simulink model "EVX_Lap_Simulation 2"  (R2018b)
settings: Solver=FixedStepAuto  StartTime=0  StopTime=120  FixedStep=0.001  MaxStep=0.01  RelTol=1e-2
values from neighbouring files (symbols this model uses):
  velocity_dnew = velocity_d + 0.4 .* (velocity_dmax - velocity_d)    [Run_Sim(with_fmincon).m]
undefined symbols (not defined in the file or in its folder): dist, theta_d
libraries: simulink x1
(part 3 of 3)

== matlab function EVX_Lap_Simulation 2/EVX_Vehicle_Model/Car_Parameters/MATLAB Function20 ==
  data: Fzo output; Ro output; q_Bz1 output; q_Bz2 output; q_Bz3 output; q_Bz4 output; q_Bz5 output; q_Bz9 output; q_Bz10 output; q_Cz1 output; q_Dz1 output; q_Dz2 output; q_Dz3 output; q_Dz4 output; q_Dz6 output; q_Dz7 output; q_Dz8 output; q_Dz9 output; q_Ez1 output; q_Ez2 output; q_Ez3 output; q_Ez4 output; q_Ez5 output; q_Hz1 output; q_Hz2 output; q_Hz3 output; q_Hz4 output; p_Cy1 output; p_Dy1 output; p_Dy2 output; p_Dy3 output; p_Ey1 output; p_Ey2 output; p_Ey3 output; p_Ey4 output; p_Ky1 output; p_Ky2 output; p_Ky3 output; p_Hy1 output; p_Hy2 output; p_Hy3 output; p_Vy1 output; p_Vy2 output; p_Vy3 output; p_Vy4 output; p_Cx1 output; p_Dx1 output; p_Dx2 output; p_Ex1 output; p_Ex2 output; p_Ex3 output; p_Ex4 output; p_Kx1 output; p_Kx2 output; p_Kx3 output; p_Hx1 output; p_Hx2 output; p_Vx1 output; p_Vx2 output
function [Fzo,Ro,q_Bz1,q_Bz2,q_Bz3,q_Bz4,q_Bz5,q_Bz9,q_Bz10,q_Cz1,q_Dz1,...
    q_Dz2,q_Dz3,q_Dz4,q_Dz6,q_Dz7,q_Dz8,q_Dz9,q_Ez1,q_Ez2,q_Ez3,q_Ez4,q_Ez5,...
    q_Hz1,q_Hz2,q_Hz3,q_Hz4,p_Cy1,p_Dy1,p_Dy2,p_Dy3,p_Ey1,p_Ey2,p_Ey3,...
    p_Ey4,p_Ky1,p_Ky2,p_Ky3,p_Hy1,p_Hy2,p_Hy3,p_Vy1,p_Vy2,p_Vy3,p_Vy4,...
    p_Cx1,p_Dx1,p_Dx2,p_Ex1,p_Ex2,p_Ex3,p_Ex4,p_Kx1,p_Kx2,p_Kx3,p_Hx1,...
    p_Hx2,p_Vx1,p_Vx2] = Avon_FITO9241
% pacejka model coefficients provided by Stackpole Engineering Services
% for Avon tyre model FITO 9241
% as found in the document 'SES_FSAE_Tiredata_Rev3'
% Specs:
% Size	6.2/20-13
% Pressure 12 psi


Fzo =	1122.74; % N
Ro = 0.25400; % m

% [ALIGNING COEFFICIENTS]
q_Bz1 =	6.11547;
q_Bz2 =	-1.96461;
q_Bz3 =	1.02155;
q_Bz4 =	5.41323;
q_Bz5 =	-7.58049;
q_Bz9 =	0;
q_Bz10 = 0;
q_Cz1 =	1.25000;
q_Dz1 =	0.15275;
q_Dz2 =	-0.00637;
q_Dz3 =	-0.21282;
q_Dz4 =	0.02719;
q_Dz6 =	-0.00145;
q_Dz7 =	0.01039;
q_Dz8 =	-1.03566;
q_Dz9 =	0.24508;
q_Ez1 =	-4.00001;
q_Ez2 =	0;
q_Ez3 =	0.00003;
q_Ez4 =	0.29616;
q_Ez5 =	2.43287;
q_Hz1 =	-0.00124;
q_Hz2 =	-0.00769;
q_Hz3 =	0.49190;
q_Hz4 =	0.13660;

%  [LATERAL COEFFICIENTS]
p_Cy1 =	0.95232;
p_Dy1 =	2.65462;
p_Dy2 =	0.05198;
p_Dy3 =	-13.51679;
p_Ey1 =	0.29170;
p_Ey2 =	0.30617;
p_Ey3 =	-0.53331;
p_Ey4 =	1.52410;
p_Ky1 =	-27.31900;
p_Ky2 =	-1.06469;
p_Ky3 =	2.27460;
p_Hy1 =	0.00227;
p_Hy2 =	-0.00772;
p_Hy3 =	-0.12814;
p_Vy1 =	0.14237;
p_Vy2 =	-0.17287;
p_Vy3 =	-1.49583;
p_Vy4 =	4.55061;

% [LONGITUDINAL COEFFICIENTS]
p_Cx1 = 1.43990;
p_Dx1 =	2.59060;
p_Dx2 =	-0.36627;
p_Ex1 =	-0.24355;
p_Ex2 =	-0.66953;
p_Ex3 =	-3.71110;
p_Ex4 =	0.37836;
p_Kx1 =	36.76960;
p_Kx2 =	-23.37320;
p_Kx3 =	-0.45230;
p_Hx1 =	0.00098;
p_Hx2 =	0.00014;
p_Vx1 =	-0.04913;
p_Vx2 =	0.02482;

== matlab function EVX_Lap_Simulation 2/EVX_Vehicle_Model/Subsystem1/MATLAB Function8 ==
  data: Fz input; Fxo output; kappa input; alpha input; gam input; Fzo input; Ro input; Fyo output; Mzo output; q_Bz1 input; q_Bz2 input; q_Bz3 input; q_Bz4 input; q_Bz5 input; q_Bz9 input; q_Bz10 input; q_Cz1 input; q_Dz1 input; q_Dz2 input; q_Dz3 input; q_Dz4 input; q_Dz6 input; q_Dz7 input; q_Dz8 input; q_Dz9 input; q_Ez1 input; q_Ez2 input; q_Ez3 input; q_Ez4 input; q_Ez5 input; q_Hz1 input; q_Hz2 input; q_Hz3 input; q_Hz4 input; p_Cy1 input; p_Dy1 input; p_Dy2 input; p_Dy3 input; p_Ey1 input; p_Ey2 input; p_Ey3 input; p_Ey4 input; p_Ky1 input; p_Ky2 input; p_Ky3 input; p_Hy1 input; p_Hy2 input; p_Hy3 input; p_Vy1 input; p_Vy2 input; p_Vy3 input; p_Vy4 input; p_Cx1 input; p_Dx1 input; p_Dx2 input; p_Ex1 input; p_Ex2 input; p_Ex3 input; p_Ex4 input; p_Kx1 input; p_Kx2 input; p_Kx3 input; p_Hx1 input; p_Hx2 input; p_Vx1 input; p_Vx2 input; car_mu_scaling input; run_info input
function [Fxo,Fyo,Mzo] = Pacejka_Tyre_Model(Fz,kappa,alpha,gam,Fzo,Ro,...
    q_Bz1,q_Bz2,q_Bz3,q_Bz4,q_Bz5,q_Bz9,q_Bz10,q_Cz1,q_Dz1,...
    q_Dz2,q_Dz3,q_Dz4,q_Dz6,q_Dz7,q_Dz8,q_Dz9,q_Ez1,q_Ez2,q_Ez3,q_Ez4,q_Ez5,...
    q_Hz1,q_Hz2,q_Hz3,q_Hz4,p_Cy1,p_Dy1,p_Dy2,p_Dy3,p_Ey1,p_Ey2,p_Ey3,...
    p_Ey4,p_Ky1,p_Ky2,p_Ky3,p_Hy1,p_Hy2,p_Hy3,p_Vy1,p_Vy2,p_Vy3,p_Vy4,...
    p_Cx1,p_Dx1,p_Dx2,p_Ex1,p_Ex2,p_Ex3,p_Ex4,p_Kx1,p_Kx2,p_Kx3,p_Hx1,...
    p_Hx2,p_Vx1,p_Vx2,car_mu_scaling,run_info)
% Pacejka '96 tyre model
%
% Inputs:
% Fz:       normal force (N)
% kappa:    slip ratio (% between -1 and 1) +ve is driving, -ve is braking
% alpha:    slip angle (rad) +ve alpha generates +ve Fyo
% gam:      inclanation angle/camber (rad) +ve indicates top of tyre tipped
%           right
% Outputs:
% Fxo:      Longitudinal force (N)
% Fyo:      Lateral force (N)
% Mzo:      Aligning moment (Nm)


%% tyre coefficients
% each different type of tyre holds different scaling coefficients, load 
% these here Also loaded are unloaded tyre radius and nominal wheel load

% unpack the structure holding the coefficients
% Get the field names of the structure
% fields = fieldnames(carpacejka_coefs, '-full');

% for ii = 1:length(fields)
%     thisField = fields{ii};
%     create_variable = sprintf('%s = carpacejka_coefs%s;', thisField, thisField);
%     eval(create_variable);
% end
% clear('ii', 'thisField');
% clear('fields', 'create_variable');

%% register track conditions
% scaling factors affected by wet/dry conditions

    lambda_mux = 1; % peak friction coefficient
    lambda_muy = 1; % peak friction coefficient

% modify with user scaling factor
lambda_mux = lambda_mux*car_mu_scaling;
lambda_muy = lambda_muy*car_mu_scaling;

%% scaling factors
% default values for these values is 1 (except lambda_muV=0)
lambda_Fzo = 1; % nominal rated load
lambda_muV = 0; % with slip speed Vx decaying friction
lambda_Kx = 1; % brake slip stiffness
lambda_Ky = 1; % cornering stiffness
lambda_Cx = 1; % shape factor
lambda_Cy = 1; % shape factor
lambda_Ex = 1; % curvature factor
lambda_Ey = 1; % curvature factor
lambda_Hx = 1; % horizontal shift
lambda_Hy = 1; % horizontal shift
lambda_Vx = 1; % vertical shift
lambda_Vy = 1; % vertical shift
lambda_Kygam = 1; % camber force stiffness
lambda_Kzgam = 1; % camber torque stiffness
lambda_t = 1; % pneumatic trail
lambda_Mr = 1; % residual torque
lambda_ygam = 1;

if ~isrow(kappa) || ~isrow(alpha) || ~isrow(gam)
    kappa = transpose(kappa);
    alpha = transpose(alpha);
    gam = transpose(gam);
end

for ii=1:length(Fz)
    %% derived inputs
    dfz = (Fz(ii)-Fzo)/Fzo; % normalised change in vertical load
    
    %% longitudinal force (pure longitudinal slip)
    S_Vx = Fz(ii)*(p_Vx1+p_Vx2*dfz)*lambda_Vx*lambda_mux;
    S_Hx = (p_Hx1+p_Hx2*dfz)*lambda_Hx;
    kappa_x = kappa + S_Hx;
    K_xk = Fz(ii)*(p_Kx1+p_Kx2*dfz)*exp(-p_Kx3*dfz)*lambda_Kx;
    E_x = (p_Ex1+p_Ex2*dfz+p_Ex3*dfz^2)*(1-p_Ex4*sign(kappa_x))*lambda_Ex;
    mu_x = (p_Dx1+p_Dx2*dfz)*lambda_mux;
    D_x = mu_x*Fz(ii);
    C_x = p_Cx1*lambda_Cx;
    B_x = K_xk/(C_x*D_x);
    Fxo = D_x*sin(C_x*atan(B_x*kappa_x - E_x*(B_x*kappa_x-atan(B_x*kappa_x)))) + S_Vx;
    
    %% lateral force (pure lateral slip)
    gam_y = gam*lambda_ygam;
    C_y = p_Cy1*lambda_Cy;
    mu_y = (p_Dy1+p_Dy2*dfz)*(1-p_Dy3*gam^2)*lambda_muy;
    D_y = mu_y*Fz(ii);
    S_Hy = (p_Hy1+p_Hy2*dfz+p_Hy3*gam)*lambda_Hy;
    alpha_y = alpha + S_Hy;
    E_y = (p_Ey1+p_Ey2*dfz)*(1-(p_Ey3+p_Ey4*gam_y)*sign(alpha_y))*lambda_Ey;
    K_ya = p_Ky1*Fzo*sin(2*atan(Fz(ii)/(p_Ky2*Fzo*lambda_Fzo)))*(1-p_Ky3*abs(gam))*lambda_Fzo*lambda_Ky;
    B_y = K_ya/(C_y*D_y);
    S_Vy = Fz(ii)*((p_Vy1+p_Vy2*dfz)+(p_Vy3+p_Vy4*dfz)*gam*lambda_Vy*lambda_Kygam);
    Fyo = D_y*sin(C_y*atan(B_y*alpha_y - E_y*(B_y*alpha_y-atan(B_y*alpha_y)))) + S_Vy;
    
    %% aligning torque (pure side slip)
    B_t = (q_Bz1+q_Bz2*dfz+q_Bz3*dfz^2)*(1+q_Bz4*gam*q_Bz5*abs(gam))*lambda_Ky/lambda_muy;
    C_t = q_Cz1;
    D_t = (q_Dz1+q_Dz2*dfz)*(1+q_Dz3*gam+q_Dz4*gam^2)*Ro*lambda_t/Fzo;
    S_Ht = q_Hz1+q_Hz2*dfz+(q_Hz3+q_Hz4*dfz)*gam;
    alpha_t = alpha + S_Ht;
    E_t = (q_Ez1+q_Ez2*dfz+q_Ez3*dfz^2)*(1+(q_Ez4+q_Ez5*gam)*atan(B_t*C_t*alpha_t));
    B_r = (q_Bz9*lambda_Ky/lambda_muy+q_Bz10*B_y*C_y);
    D_r = Fz(ii)*((q_Dz6+q_Dz7*dfz)+(q_Dz8+q_Dz9*dfz)*gam)*Ro*lambda_muy*lambda_Mr;
    S_Hf = S_Hy + S_Vy/K_ya;
    alpha_r = alpha + S_Hf;
    Mzr = D_r*cos(atan(B_r*alpha_r))*cos(alpha);
    t = D_t*cos(C_t*atan(B_t*alpha_t-E_t*(B_t*alpha_t-atan(B_t*alpha_t))))*cos(alpha);
    Mzo = -t*Fyo + Mzr;
    
end

== matlab function EVX_Lap_Simulation 2/EVX_Vehicle_Model/Subsystem1/MATLAB Function ==
  data: x input; F_z output; xdot input; k input; c input
function F_z = fcn(x,xdot,k,c)

F_z = k * x + c * xdot;

== matlab function EVX_Lap_Simulation 2/EVX_Vehicle_Model/Car_Parameters/MATLAB Function21 ==
  data: whatever input; k_SFR output; Owen input; wants input; k_SFL output; k_SRR output; k_SRL output; c_SFR output; c_SFL output; c_SRR output; c_SRL output; k_TFR output; k_TFL output; k_TRR output; k_TRL output; c_TFR output; c_TFL output; c_TRR output; c_TRL output; k_RF output; k_RR output; k_FRIC output; c_RF output; c_RR output; c_FRIC output; gamma_FR output; gamma_FL output; gamma_RR output; gamma_RL output; I_WFR output; I_WFL output; I_WRR output; I_WRL output
function [k_SFR,k_SFL,k_SRR,k_SRL,c_SFR,c_SFL,c_SRR,c_SRL,k_TFR,k_TFL,...
    k_TRR,k_TRL,c_TFR,c_TFL,c_TRR,c_TRL,k_RF,k_RR,k_FRIC,c_RF,c_RR,...
    c_FRIC,gamma_FR,gamma_FL,gamma_RR,gamma_RL,I_WFR,I_WFL,I_WRR,I_WRL]...
    = Suspension_Mapping(whatever,Owen,wants)

% Suspension Stifnesses
k_SFR = 8000; %suspension stiffness front right (N/m)
k_SFL = 8000; %suspension stiffness front left (N/m)
k_SRR = 8000; %suspension stiffness rear right (N/m)
k_SRL = 8000; %suspension stiffness rear left (N/m)

% Tire Stifnesses
k_TFR = 10000; %tire stiffness front right (N/m)
k_TFL = 10000; %tire stiffness front left (N/m)
k_TRR = 10000; %tire stiffness rear right (N/m)
k_TRL = 10000; %tire stiffness rear left (N/m)

% Suspension Damping Coefficients
c_SFR = 1000; %suspension damping coefficient front right (Ns/m)
c_SFL = 1000; %suspension damping coefficient front left (Ns/m)
c_SRR = 1000; %suspension damping coefficientv rear right (Ns/m)
c_SRL = 1000; %suspension damping coefficient rear left (Ns/m)

% Tire Damping Coefficients
c_TFR = 2000; %tire damping coefficient front right (Ns/m)
c_TFL = 2000; %tire damping coefficient front left (Ns/m)
c_TRR = 2000; %tire damping coefficientv rear right (Ns/m)
c_TRL = 2000; %tire damping coefficient rear left (Ns/m)

% Roll Bar Stiffnesses
k_RF = 0; %front
k_RR = 0; %rear
k_FRIC = 0; %front to rear

% Roll Bar Damping
c_RF = 0; %front
c_RR = 0; %rear
c_FRIC = 0; %front to rear

% Camber (deg) (tilt right positive)
gamma_FRd = 0;
gamma_FLd = 0;
gamma_RRd = 0;
gamma_RLd = 0;

% Camber (Rad)
Deg2Rad = 0.0174533;
gamma_FR = gamma_FRd * Deg2Rad;
gamma_FL = gamma_FLd * Deg2Rad;
gamma_RR = gamma_RRd * Deg2Rad;
gamma_RL = gamma_RLd * Deg2Rad;

% Wheel Inertias
I_WFR = 2;
I_WFL = 2;
I_WRR = 2;
I_WRL = 2;

== matlab function EVX_Lap_Simulation 2/EVX_Vehicle_Model/MATLAB Function22 ==
  data: g output
function g  = Environment_Parameters

g = 9.81;

== matlab function EVX_Lap_Simulation 2/EVX_Vehicle_Model/Chassis Vertical Dynamics/MATLAB Function22 ==
  data: g input; F_zWFR output; m_WFR input; m_WFL input; m_WRR input; m_WRL input; F_zWFL output; F_zWRR output; F_zWRL output
function [F_zWFR,F_zWFL,F_zWRR,F_zWRL] = fcn(g,m_WFR,m_WFL,m_WRR,m_WRL)

F_zWFR = -g * m_WFR;
F_zWFL = -g * m_WFL;
F_zWRR = -g * m_WRR;
F_zWRL = -g * m_WRL;

== matlab function EVX_Lap_Simulation 2/EVX_Vehicle_Model/MATLAB Function23 ==
  data: v_y input; ratio_FR output; angle_FR output; ratio_FL output; angle_FL output; ratio_RR output; angle_RR output; ratio_RL output; angle_RL output; v_x input; a input; b input; d_F input; e_F input; d_R input; e_R input; Idot_z input; r_FR input; r_FL input; r_RR input; r_RL input; S_FR input; S_FL input; S_RR input; S_RL input; w_FR input; w_FL input; w_RR input; w_RL input
function [ratio_FR,angle_FR,ratio_FL,angle_FL,ratio_RR,angle_RR,ratio_RL,...
    angle_RL] = Tyre_Slips(v_y,v_x,a,b,d_F,e_F,d_R,e_R,Idot_z,r_FR,r_FL,...
    r_RR,r_RL,S_FR,S_FL,S_RR,S_RL,w_FR,w_FL,w_RR,w_RL)

beta = atan(v_y/v_x);

v_yFR = v_y + Idot_z * a;
v_yFL = v_y + Idot_z * a;
v_yRR = v_y + Idot_z * -b;
v_yRL = v_y + Idot_z * -b;

v_xFR = v_x - Idot_z * e_F;
v_xFL = v_x - Idot_z * -d_F;
v_xRR = v_x - Idot_z * e_R;
v_xRL = v_x - Idot_z * -d_R;

beta_FR = atan(v_yFR/v_xFR);
beta_FL = atan(v_yFL/v_xFL);
beta_RR = atan(v_yRR/v_xRR);
beta_RL = atan(v_yRL/v_xRL);

w0_FR = v_x / r_FR;
w0_FL = v_x / r_FL;
w0_RR = v_x / r_RR;
w0_RL = v_x / r_RL;

ratio_FR = (w_FR - w0_FR)/w0_FR;
angle_FR = beta_FR - S_FR;
ratio_FL = (w_FL - w0_FL)/w0_FL;
angle_FL = beta_FL - S_FL;
ratio_RR = (w_RR - w0_RR)/w0_RR;
angle_RR = beta_RR - S_RR;
ratio_RL = (w_RL - w0_RL)/w0_RL;
angle_RL = beta_RL - S_RL;

% ratio_FR = 0;
% angle_FR = 0;
% ratio_FL = 0;
% angle_FL = 0;
% ratio_RR = 0;
% angle_RR = 0;
% ratio_RL = 0;
% angle_RL = 0;

== matlab function EVX_Lap_Simulation 2/EVX_Vehicle_Model/Aero Model/MATLAB Function ==
  data: v_x input; F_d output
function F_d = Drag(v_x)

F_d = v_x * 10;

== matlab function EVX_Lap_Simulation 2/EVX_Vehicle_Model/Tyre Model/Pacejka Tyre Model/MATLAB Function5 ==
  data: SA input; F_y output; SL input; Fz input; F_x output; M_z output
function [F_y,F_x,M_z] = Pacejka4(SA,SL,Fz)
x1  =  0.0174533 .* SA;  %Slip
x2  = Fz;  % Fz
x3  =  150 * 0.0174533 .* SL;  %Slip ratio, with fudge factor
P = [2 1 12.5 1.55]; %Fitted to FSAE TTC Round 6 Run 2
D1  = P(1);
D2  = P(2);
B   = P(3);
C   = P(4);
D   = (D1 + D2/1000 .* x2) .* x2;   % peak value (normalized)
F_y  = D .* sin(C .* atan(B .* x1));
F_x  = D .*sin (C .* atan(B .* x3));
M_z = [0 0 0 0];

== matlab function EVX_Lap_Simulation 2/EVX_Vehicle_Model/Aero Model/MATLAB Function1 ==
  data: v_x input; F_z output
function F_z = Drag(v_x)

F_z = v_x * 2;

== matlab function EVX_Lap_Simulation 2/EVX_Vehicle_Model/Tyre Model/MATLAB Function1 ==
  data: x_W input; F_zT output; xdot_W input; k_T input; c_T input
function F_zT  = fcn(x_W,xdot_W,k_T,c_T)

F_zT = k_T .* (-x_W) + c_T .* (-xdot_W);

== matlab function EVX_Lap_Simulation 2/EVX Vehicle Model V2/Vertical Dynamics/8DOF Vibrations ==
  data: V input; A output; V output; D input; F input; zB input; dzB input; D output; w input; m input; I input; kc input; cc input; kt input; ks input; kr input; ct input; cs input; cr input; kt output; ct output
function [A,V,D,kt,ct] =   DOF_Dynamics(V,D,F,zB,dzB,w,m,I,kc,cc,kt,ks,kr,ct,cs,cr)

% Tyre Stifness = 0 when off ground
for i = 1:4
    if D(i) - zB(i) > 0
        kt(i) = 0;
        ct(i) = 0;
    end
end

% Wheel Positions
x_wFL = w(1,1);
x_wFR = w(1,2);
x_wRL = w(1,3);
x_wRR = w(1,4);

y_wFL = w(2,1);
y_wFR = w(2,2);
y_wRL = w(2,3);
y_wRR = w(2,4);

% Chassis Forces
Fw_FL = F(1);
Fw_FR = F(2);
Fw_RL = F(3);
Fw_RR = F(4);
Fc_z = F(5);
Mc_y = F(6);
McF_x = F(7);
McR_x = F(8);

% Mass & Intertias
m_WFL = m(1);
m_WFR = m(2);
m_WRL = m(3);
m_WRR = m(4);
m_c = m(5);
I_cy = I(1);
I_xF = I(2);
I_xR = I(3);
I_z = I(4);

% Base Displacements
zB_FL = zB(1);
zB_FR = zB(2);
zB_RL = zB(3);
zB_RR = zB(4);

% Base Velocities
dzB_FL = dzB(1);
dzB_FR = dzB(2);
dzB_RL = dzB(3);
dzB_RR = dzB(4);

% Tyre Stiffness
kt_FL = kt(1);
kt_FR = kt(2);
kt_RL = kt(3);
kt_RR = kt(4);

% Suspension Stiffness
ks_FL = ks(1);
ks_FR = ks(2);
ks_RL = ks(3);
ks_RR = ks(4);

% Rollbar Stiffness
kr_Fx = kr(1);
kr_Rx = kr(2);
kr_Ly = kr(3);
kr_Ry = kr(4);
kr_FLRR = kr(5);
kr_FRRL = kr(6);

% Chassis Stiffness
kc_x = kc(1);

% Tyre Damping
ct_FL = ct(1);
ct_FR = ct(2);
ct_RL = ct(3);
ct_RR = ct(4);

% Suspension Damping
cs_FL = cs(1);
cs_FR = cs(2);
cs_RL = cs(3);
cs_RR = cs(4);

% Rollbar Damping
cr_Fx = cr(1);
cr_Rx = cr(2);
cr_Ly = cr(3);
cr_Ry = cr(4);
cr_FLRR = cr(5);
cr_FRRL = cr(6);

% Chassis Damping
cc_x = cc(1);

% Displacements
z_wFL = D(1);
z_wFR = D(2);
z_wRL = D(3);
z_wRR = D(4);
z_c = D(5);
thetay_c = D(6);
thetax_F = D(7);
thetax_R = D(8);

% Velocities
dz_wFL = V(1);
dz_wFR = V(2);
dz_wRL = V(3);
dz_wRR = V(4);
dz_c = V(5);
dthetay_c = V(6);
dthetax_F = V(7);
dthetax_R = V(8);

% Accelerations

ddz_wFL = (1 / m(1)) * (F(1)...
    + kt(1) * (zB(1) - D(1))...
    - ks(1) * (D(1) - D(5) + w(1,1) * D(6) - w(2,1) * D(7))...
    + ct(1) * (dzB(1) - V(1))...
    - cs(1) * (V(1) - V(5) + w(1,1) * V(6) - w(2,1) * V(7))...
    + kr(1) * (D(2) - D(1))...
    - kr(3) * (D(1) - D(3))...
    - kr(5) * (D(1) - D(4))...
    + cr(1) * (V(2) - V(1))...
    - cr(3) * (V(1) - V(3))...
    - cr(5) * (V(1) - V(4)));

ddz_wFR = (1 / m(2)) * (F(2)...
    + kt(2) * (zB(2) - D(2))...
    - ks(2) * (D(2) - D(5) + w(1,2) * D(6) - w(2,2) * D(7))...
    + ct(2) * (dzB(2) - V(2))...
    - cs(2) * (V(2) - V(5) + w(1,2) * V(6) - w(2,2) * V(7))...
    - kr(1) * (D(2) - D(1))...
    - kr(4) * (D(2) - D(4))...
    - kr(6) * (D(2) - D(3))...
    - cr(1) * (V(2) - V(1))...
    - cr(4) * (V(2) - V(4))...
    - cr(6) * (V(2) - V(3)));

ddz_wRL = (1 / m(3)) * (F(3)...
    + kt(3) * (zB(3) - D(3))...
    - ks(3) * (D(3) - D(5) + w(1,3) * D(6) - w(2,3) * D(8))...
    + ct(3) * (dzB(3) - V(3))...
    - cs(3) * (V(3) - V(5) + w(1,3) * V(6) - w(2,3) * V(8))...
    + kr(2) * (D(4) - D(3))...
    + kr(3) * (D(1) - D(3))...
    + kr(6) * (D(2) - D(3))...
    + cr(2) * (V(4) - V(3))...
    + cr(3) * (V(1) - V(3))...
    + cr(6) * (V(2) - V(3)));

ddz_wRR = (1 / m(4)) * (F(4)...
    + kt(4) * (zB(4) - D(4))...
    - ks(4) * (D(4) - D(5) + w(1,4) * D(6) - w(2,4) * D(8))...
    + ct(4) * (dzB(4) - V(4))...
    - cs(4) * (V(4) - V(5) + w(1,4) * V(6) - w(2,4) * V(8))...
    - kr(2) * (D(4) - D(3))...
    + kr(4) * (D(2) - D(4))...
    + kr(5) * (D(1) - D(4))...
    - cr(2) * (V(4) - V(3))...
    + cr(4) * (V(2) - V(4))...
    + cr(5) * (V(1) - V(4)));

ddz_c = (1 / m(5)) * (F(5)...
    + ks(1) * (D(1) - D(5) + w(1,1) * D(6) - w(2,1) * D(7))...
    + ks(2) * (D(2) - D(5) + w(1,2) * D(6) - w(2,2) * D(7))...
    + ks(3) * (D(3) - D(5) + w(1,3) * D(6) - w(2,3) * D(8))...
    + ks(4) * (D(4) - D(5) + w(1,4) * D(6) - w(2,4) * D(8))...
    + cs(1) * (V(1) - V(5) + w(1,1) * V(6) - w(2,1) * V(7))...
    + cs(2) * (V(2) - V(5) + w(1,2) * V(6) - w(2,2) * V(7))...
    + cs(3) * (V(3) - V(5) + w(1,3) * V(6) - w(2,3) * V(8))...
    + cs(4) * (V(4) - V(5) + w(1,4) * V(6) - w(2,4) * V(8)));

ddthetay_c = (1 / I(1)) * (F(6)...
    - w(1,1) * ks(1) * (D(1) - D(5) + w(1,1) * D(6) - w(2,1) * D(7))...
    - w(1,2) * ks(2) * (D(2) - D(5) + w(1,2) * D(6) - w(2,2) * D(7))...
    - w(1,3) * ks(3) * (D(3) - D(5) + w(1,3) * D(6) - w(2,3) * D(8))...
    - w(1,4) * ks(4) * (D(4) - D(5) + w(1,4) * D(6) - w(2,4) * D(8))...
    - w(1,1) * cs(1) * (V(1) - V(5) + w(1,1) * V(6) - w(2,1) * V(7))...
    - w(1,2) * cs(2) * (V(2) - V(5) + w(1,2) * V(6) - w(2,2) * V(7))...
    - w(1,3) * cs(3) * (V(3) - V(5) + w(1,3) * V(6) - w(2,3) * V(8))...
    - w(1,4) * cs(4) * (V(4) - V(5) + w(1,4) * V(6) - w(2,4) * V(8)));

dthetax_F = (1 / I(2)) * (F(7)...
    + w(2,1) * ks(1) * (D(1) - D(5) + w(1,1) * D(6) - w(2,1) * D(7))...
    + w(2,2) * ks(2) * (D(2) - D(5) + w(1,2) * D(6) - w(2,2) * D(7))...
    - kc(1) * (D(7) - D(8))...
    + w(2,1) * cs(1) * (V(1) - V(5) + w(1,1) * V(6) - w(2,1) * V(7))...
    + w(2,2) * cs(2) * (V(2) - V(5) + w(1,2) * V(6) - w(2,2) * V(7))...
    - cc(1) * (V(7) - V(8)));

ddthetax_R = (1 / I(3)) * (F(8)...
	+ w(2,3) * ks(3) * (D(3) - D(5) + w(1,3) * D(6) - w(2,3) * D(8))...
    + w(2,4) * ks(4) * (D(4) - D(5) + w(1,4) * D(6) - w(2,4) * D(8))...
    + kc(1) * (D(7) - D(8))...
	+ w(2,3) * cs(3) * (V(3) - V(5) + w(1,3) * V(6) - w(2,3) * V(8))...
    + w(2,4) * cs(4) * (V(4) - V(5) + w(1,4) * V(6) - w(2,4) * V(8))...
    + cc(1) * (D(7) - D(8)));

A = [ddz_wFL;ddz_wFR;ddz_wRL;ddz_wRR;ddz_c;ddthetay_c;dthetax_F;ddthetax_R];

== matlab function EVX_Lap_Simulation 2/EVX Vehicle Model V2/Horizontal Dynamics/Tyre_Forces ==
  data: F_TxFL input; F_x output; F_TxFR input; F_TxRL input; F_TxRR input; F_TyFL input; F_TyFR input; F_TyRL input; F_TyRR input; M_TzFL input; M_TzFR input; M_TzRL input; M_TzRR input; S input; w input; F_y output; M_z output
function [F_x,F_y,M_z] = Tyre_Forces(F_TxFL,F_TxFR,F_TxRL,F_TxRR...
    ,F_TyFL,F_TyFR,F_TyRL,F_TyRR,M_TzFL,M_TzFR,M_TzRL,M_TzRR,S,w)

F_TyRL = -F_TyRL;
F_TyRR = -F_TyRR;

F_x = F_TxFL * cosd(S(1)) - F_TyFL * sind(S(1))...
    + F_TxFR * cosd(S(2)) - F_TyFR * sind(S(2))...
    + F_TxRL * cosd(S(3)) - F_TyRL * sind(S(3))...
    + F_TxRR * cosd(S(4)) - F_TyRR * sind(S(4));

F_y = F_TxFL * sind(S(1)) + F_TyFL * cosd(S(1))...
    + F_TxFR * sind(S(2)) + F_TyFR * cosd(S(2))...
    - F_TxRL * sind(S(3)) - F_TyRL * cosd(S(3))...
    - F_TxRR * sind(S(4)) - F_TyRR * cosd(S(4));

M_z = F_TxFL * (w(1,1) * sind(S(1)) - w(2,1) * cosd(S(1)))...
    + F_TyFL * (w(2,1) * sind(S(1)) + w(1,1) * cosd(S(1)))...
    + F_TxFR * (w(1,2) * sind(S(2)) - w(2,2) * cosd(S(2)))...
    + F_TyFR * (w(2,2) * sind(S(2)) + w(1,2) * cosd(S(2)))...
    + F_TxRL * (-w(1,3) * sind(S(3)) - w(2,3) * cosd(S(3)))...
    + F_TyRL * (w(2,3) * sind(S(3)) - w(1,3) * cosd(S(3)))...
    + F_TxRR * (-w(1,4) * sind(S(4)) - w(2,4) * cosd(S(4)))...
    + F_TyRR * (w(2,4) * sind(S(4)) - w(1,4) * cosd(S(4)))...
    - M_TzFL - M_TzFR + M_TzRL + M_TzRR;

== matlab function EVX_Lap_Simulation 2/EVX Vehicle Model V2/Aero Model/Forces ==
  data: v_x input; F_L output; F_D output
function [F_L,F_D] = fcn(v_x)

F_L = 10 * v_x^2;
F_D = 5 * v_x^2;

== matlab function EVX_Lap_Simulation 2/EVX Vehicle Model V2/Vertical Dynamics/MATLAB Function2 ==
  data: t input; zB output
function zB = fcn(t)

% Base Displacements

% zB_FL = 0;
% zB_FR = 0;
% zB_RL = 0;
% zB_RR = 0;
% 
% if t > 2
%     zB_FL = 0.01;
%     zB_RL = 0.00;
% end
% 
% if t > 3
%     zB_FL = 0.01;
%     zB_RL = 0.01;
% end
% 
% if t > 4
%     zB_FL = 0.015;
%     zB_RL = 0.015;
% end
% 
% if t > 5
%     zB_FL = 0;
%     zB_RL = 0;
% end
% 
% if t > 7
% zB_FL = 0.001 * sin(2*t);
% zB_FR = -0.001 * sin(2*t);
% zB_RL = 0.001 * sin(2*t);
% zB_RR = -0.001 * sin(2*t);
% end
% 
% if t > 15
% zB_FL = 0.001 * sin(3*t) - 0.005;
% zB_FR = -0.001 * sin(3*t);
% zB_RL = 0.001 * sin(3*t) - 0.005;
% zB_RR = -0.001 * sin(3*t);
% end

zB_FL = 0;
zB_FR = 0;
zB_RL = 0;
zB_RR = 0;

zB = [zB_FL,zB_FR,zB_RL,zB_RR];

== matlab function EVX_Lap_Simulation 2/EVX Vehicle Model V2/Vertical Dynamics/MATLAB Function3 ==
  data: V output; F input; zB input; D output; w input; kc input; kt input; ks input; kr input
function [V,D] = Initial_SS(F,zB,w,kc,kt,ks,kr)

% syms z_WFL z_WFR z_WRL z_WRR z_c thetay thetax_F thetax_R
% 
% eq_FL = F(1) + zB(1) * kt(1)...
% 	== z_WFL * (kt(1) + ks(1) + kr(1) + kr(3) + kr(5))...
% 	 + z_WFR * (-kr(1))...
%      + z_WRL * (-kr(2))...
%      + z_wRR * (-kr(5))...
%      + z_c * (-ks(1))...
%      + thetay * (w(1,1) * ks(1))...
%      + thetax_F * (-w(2,1) * ks(1))...
%      + thetax_R * (0);
%  
% eq_FR = F(2) + zB(2) * kt(2)...
% 	== z_WFL * (-kr(1))...
% 	 + z_WFR * (kt(2) + ks(2) + kr(1) + kr(4) + kr(6))...
%      + z_WRL * (-kr(6))...
%      + z_wRR * (-kr(4))...
%      + z_c * (-ks(2))...
%      + thetay * (w(1,2) * ks(2))...
%      + thetax_F * (-w(2,2) * ks(2))...
%      + thetax_R * (0);
% 
% eq_RL = F(3) + zB(3) * kt(3)...
% 	== z_WFL * (-kr(3))...
% 	 + z_WFR * (-kr(6))...
%      + z_WRL * (kt(3) + ks(3) + kr(2) + kr(3) + kr(6))...
%      + z_wRR * (-kr(2))...
%      + z_c * (-ks(3))...
%      + thetay * (w(1,3) * ks(3))...
%      + thetax_F * (0)...
%      + thetax_R * (-w(2,3) * ks(3));
%  
% eq_RR = F(4) + zB(4) * kt(4)...
% 	== z_WFL * (-kr(5))...
% 	 + z_WFR * (-kr(4))...
%      + z_WRL * (-kr(2))...
%      + z_wRR * (kt(4) + ks(4) + kr(2) + kr(4) + kr(5))...
%      + z_c * (-ks(4))...
%      + thetay * (w(1,4) * ks(4))...
%      + thetax_F * (0)...
%      + thetax_R * (-w(2,4) * ks(4));
%  
% eq_zc = F(5)...
%     == z_WFL * (-ks(1))...
%      + z_WFR * (-ks(2))...
%      + z_WRL * (-ks(3))...
%      + z_WRR * (-ks(4))...
%      + z_c * (ks(1) + ks(2) + ks(3) + ks(4))...
%      + thetay * (-W(1,1) * ks(1) - w(1,2) * ks(2) - w(1,3) * ks(3) - w(1,4) * ks(4))...
%      + thetax_F * (w(2,1) * ks(1) + w(2,2) * ks(2))...
%      + thetax_R * (w(2,3) * ks(3) + w(2,4) * ks(4));
%  
% eq_thetay = F(6)...
%     == z_WFL * (w(1,1) * ks(1))...
%      + z_WFR * (w(1,2) * ks(2))...
%      + z_WRL * (w(1,3) * ks(3))...
%      + z_WRR * (w(1,4) * ks(4))...
%      + z_c * (-w(1,1) * ks(1) - w(1,2) * ks(2) - w(1,3) * ks(3) - w(1,4) * ks(4))...
%      + thetay * ((w(1,1))^2 * ks(1) + (w(1,2))^2 * ks(2) + (w(1,3))^2 * ks(3) + (w(1,4))^2 * ks(4))...
%      + thetax_F * (-w(1,1) * w(2,1) * ks(1) - w(1,2) * w(2,2) * ks(2))...
%      + thetax_R * (-w(1,3) * w(2,3) * ks(3) - w(1,4) * w(2,4) * ks(4));
%  
% eq_thetax_F = F(7)...
%     == z_WFL * (-w(2,1) * ks(1))...
%      + z_WFR * (-w(2,2) * ks(2))...
%      + z_WRL * (0)...
%      + z_WRR * (0)...
%      + z_c * (w(2,1) * ks(1) + w(2,2) * ks(2))...
%      + thetay * (-w(1,1) * w(2,1) * ks(1) - w(1,2) * w(2,2) * ks(2))...
%      + thetax_F * ((w(2,1))^2 * ks(1) + (w(2,2))^2 * ks(2) + kc(1))...
%      + thetax_R * (-kc(1));
% 
% eq_thetax_R = F(8)...
%     == z_WFL * (0)...
%      + z_WFR * (0)...
%      + z_WRL * (-w(2,3) * ks(3))...
%      + z_WRR * (-w(2,4) * ks(4))...
%      + z_c * (w(2,3) * ks(3) + w(2,4) * ks(4))...
%      + thetay * (-w(1,3) * w(2,3) * ks(3) - w(1,4) * w(2,4) * ks(4))...
%      + thetax_F * (-kc(1))...
%      + thetax_R * ((w(2,3))^2 * ks(3) + (w(2,4))^2 * ks(4) + kc(1));
%  
% [F,k] = equationsToMatrix([eq_FL,eq_FR,eq_RL,eq_RR,eq_zc,eq_thetay,eq_thetax_F,eq_thetax_R]);

% Force = [F(1) + zB(1) * kt(1);F(2) + zB(2) * kt(2);F(3) + zB(3) * kt(3);...
%     F(4) + zB(4) * kt(4);F(5);F(6);F(7);F(8)];

k1 = [(kt(1) + ks(1) + kr(1) + kr(3) + kr(5)),...
	 (-kr(1)),...
     (-kr(3)),...
     (-kr(5)),...
     (-ks(1)),...
     (w(1,1) * ks(1)),...
     (-w(2,1) * ks(1)),...
     (0)];
 
k2 = [(-kr(1)),...
	 (kt(2) + ks(2) + kr(1) + kr(4) + kr(6)),...
     (-kr(6)),...
     (-kr(4)),...
     (-ks(2)),...
     (w(1,2) * ks(2)),...
     (-w(2,2) * ks(2)),...
     (0)];

k3 = [(-kr(3)),...
	 (-kr(6)),...
     (kt(3) + ks(3) + kr(2) + kr(3) + kr(6)),...
     (-kr(2)),...
     (-ks(3)),...
     (w(1,3) * ks(3)),...
     (0),...
     (-w(2,3) * ks(3))];
 
k4 = [(-kr(5)),...
	 (-kr(4)),...
     (-kr(2)),...
     (kt(4) + ks(4) + kr(2) + kr(4) + kr(5)),...
     (-ks(4)),...
     (w(1,4) * ks(4)),...
     (0),...
     (-w(2,4) * ks(4))];
 
k5 = [(-ks(1)),...
     (-ks(2)),...
     (-ks(3)),...
     (-ks(4)),...
     (ks(1) + ks(2) + ks(3) + ks(4)),...
     (-w(1,1) * ks(1) - w(1,2) * ks(2) - w(1,3) * ks(3) - w(1,4) * ks(4)),...
     (w(2,1) * ks(1) + w(2,2) * ks(2)),...
     (w(2,3) * ks(3) + w(2,4) * ks(4))];
 
k6 = [(w(1,1) * ks(1)),...
     (w(1,2) * ks(2)),...
     (w(1,3) * ks(3)),...
     (w(1,4) * ks(4)),...
     (-w(1,1) * ks(1) - w(1,2) * ks(2) - w(1,3) * ks(3) - w(1,4) * ks(4)),...
     ((w(1,1))^2 * ks(1) + (w(1,2))^2 * ks(2) + (w(1,3))^2 * ks(3) + (w(1,4))^2 * ks(4)),...
     (-w(1,1) * w(2,1) * ks(1) - w(1,2) * w(2,2) * ks(2)),...
     (-w(1,3) * w(2,3) * ks(3) - w(1,4) * w(2,4) * ks(4))];
 
k7 = [(-w(2,1) * ks(1)),...
     (-w(2,2) * ks(2)),...
     (0),...
     (0),...
     (w(2,1) * ks(1) + w(2,2) * ks(2)),...
     (-w(1,1) * w(2,1) * ks(1) - w(1,2) * w(2,2) * ks(2)),...
     ((w(2,1))^2 * ks(1) + (w(2,2))^2 * ks(2) + kc(1)),...
     (-kc(1))];

k8 = [(0),...
     (0),...
     (-w(2,3) * ks(3)),...
     (-w(2,4) * ks(4)),...
     (w(2,3) * ks(3) + w(2,4) * ks(4)),...
     (-w(1,3) * w(2,3) * ks(3) - w(1,4) * w(2,4) * ks(4)),...
     (-kc(1)),...
     ((w(2,3))^2 * ks(3) + (w(2,4))^2 * ks(4) + kc(1))];

% D = linsolve(F,k);

k = [k1;k2;k3;k4;k5;k6;k7;k8];

D = (F/k)';

V = [0;0;0;0;0;0;0;0];

== matlab function EVX_Lap_Simulation 2/EVX Vehicle Model V2/Vertical Dynamics/MATLAB Function5 ==
  data: D input; F_T output; V input; kt input; ct input
function F_T  = Tyre_Forces(D,V,kt,ct)

D = D(1:4,:);
V = V(1:4,:);

F_T = D .* kt + V .* ct;

F_T(F_T > 0) = 0;

== matlab function EVX_Lap_Simulation 2/EVX Vehicle Model V2/Aero Model/Position ==
  data: v_x input; L output; D output
function [L,D] = fcn(v_x)

L_x = 0.8;
L_y = 0.0;
L_z = 0.5;

D_x = 0.5;
D_y = 0;
D_z = 0.4;

L = [L_x,L_y,L_z];

D = [D_x,D_y,D_z];

== matlab function EVX_Lap_Simulation 2/EVX Vehicle Model V2/Horizontal Dynamics/Aero_Forces ==
  data: F_L input; F_D input; F_x output; l input; d input; F_zC output; M_x output; M_y output; M_z output
function [F_x,F_zC,M_x,M_y,M_z] = Aero_Forces(F_L,F_D,l,d)

F_zC = -F_L;
M_x = F_L * l(2);
M_y = F_L * l(1);

F_x = -F_D;
M_y = M_y + -F_D * d(3);
M_z = F_D * d(2);

== matlab function EVX_Lap_Simulation 2/EVX Vehicle Model V2/Horizontal Dynamics/Gravitational_Forces ==
  data: m input; F_zFL output; g input; F_zFR output; F_zRL output; F_zRR output; F_zC output
function [F_zFL,F_zFR,F_zRL,F_zRR,F_zC] = Grav_Forces(m,g)

F_zFL = g * m(1);
F_zFR = g * m(2);
F_zRL = g * m(3);
F_zRR = g * m(4);
F_zC = g * m(5);

% F = [F_zFL,F_zFR,F_zRL,F_zRR,F_zC];

== matlab function EVX_Lap_Simulation 2/EVX Vehicle Model V2/Horizontal Dynamics/F=ma ==
  data: F_x input; a_x output; F_y input; M_z input; m input; I input; a_y output; ddtheta_z output
function [a_x,a_y,ddtheta_z] = F_ma(F_x,F_y,M_z,m,I)

mass = m(1) + m(2) + m(3) + m(4) + m(5);

a_x = F_x / mass;
a_y = F_y / mass;
ddtheta_z = M_z / I(4);

== matlab function EVX_Lap_Simulation 2/EVX Vehicle Model V2/Steering/Front//Rear Split ==
  data: Angle input; Steering_F output; Steering_R output
function [Steering_F,Steering_R] = Steering_Split(Angle)

Steering_F = Angle;
Steering_R = 0;

== matlab function EVX_Lap_Simulation 2/EVX Vehicle Model V2/Steering/MATLAB Function ==
  data: S_FL output; Steering_F input; S_FR output; Ratio input
function [S_FL,S_FR] = Steeting_Front(Steering_F,Ratio)

S_FL = Steering_F / Ratio;
S_FR = Steering_F / Ratio;
% 
% if abs(Steering_F) > Ratio/2
%     S_FL = S_FL + 0.5;
%     S_FR = S_FR - 0.5;
% end
%

== matlab function EVX_Lap_Simulation 2/EVX Vehicle Model V2/Steering/MATLAB Function1 ==
  data: S_RL output; Steering_R input; S_RR output; Ratio input
function [S_RL,S_RR] = Steeting_Rear(Steering_R,Ratio)

S_RL = Steering_R / Ratio;
S_RR = Steering_R / Ratio;

== matlab function EVX_Lap_Simulation 2/EVX Vehicle Model V2/Horizontal Dynamics/Position Conversion ==
  data: L input; l output; D input; w input; d output; h input
function [l,d] = fcn(L,D,w,h)

l_x = w(1) - L(1);
l_y = L(2)-((w(2,1) - w(2,2))/2 - w(2,1));
l_z = L(3) - h(1);

l = [l_x,l_y,l_z];

d_x = w(1) - D(1);
d_y = D(2)-((w(2,1) - w(2,2))/2 - w(2,1));
d_z = D(3) - h(1);

d = [d_x,d_y,d_z];

== matlab function EVX_Lap_Simulation 2/EVX Vehicle Model V2/Horizontal Dynamics/MATLAB Function ==
  data: M_x input; M_xF output; M_xR output
function [M_xF,M_xR] = fcn(M_x)

M_xF = 0.5 * M_x;
M_xR = 0.5 * M_x;

== matlab function EVX_Lap_Simulation 2/EVX Vehicle Model V2/Tyre Model/Wheel Horizontal Velocities ==
  data: v_x input; v_y input; v_xw output; dtheta_z input; w input; v_yw output
function [v_xw,v_yw] = Wheel_Velocities(v_x,v_y,dtheta_z,w)

% Wheel velocities in x direction
v_xFL = v_x - dtheta_z * w(2,1);
v_xFR = v_x - dtheta_z * w(2,2);
v_xRL = v_x - dtheta_z * w(2,3);
v_xRR = v_x - dtheta_z * w(2,4);

% Wheel velocities in y direction
v_yFL = v_y + dtheta_z * w(1,1);
v_yFR = v_y + dtheta_z * w(1,2);
v_yRL = v_y + dtheta_z * w(1,3);
v_yRR = v_y + dtheta_z * w(1,4);

v_xw = [v_xFL;v_xFR;v_xRL;v_xRR];
v_yw = [v_yFL;v_yFR;v_yRL;v_yRR];

== matlab function EVX_Lap_Simulation 2/EVX Vehicle Model V2/Wheel Dynamics/Wheel Acceleration ==
  data: F_x input; T input; I input; ddwheel output; r input
function ddwheel   = Wheel_Acceleration(F_x,T,I,r)


ddwheel = (T - (F_x .* r))./I;

== matlab function EVX_Lap_Simulation 2/EVX Vehicle Model V2/Powertrain/Motor Fucntion ==
  data: Pedal input; Torque output; Motor_Speed input; Direction input
function Torque  = Motor(Pedal,Motor_Speed,Direction)

if Pedal > 100
    Pedal = 100;
elseif Pedal < 0
    Pedal = 0;
end

power = 80000;

max_torque = 240;

torque_line = abs(power / Motor_Speed) * Direction;

Torque = min(max_torque,torque_line) * (Pedal / 100);

== matlab function EVX_Lap_Simulation 2/EVX Vehicle Model V2/Powertrain/Reverse Transmission Function ==
  data: Ratio input; Motor_Speed output; dwheel input
function Motor_Speed = Rev_Transmission(Ratio,dwheel)

Motor_Speed = ((dwheel(3) + dwheel(4)) / 2) * Ratio;

== matlab function EVX_Lap_Simulation 2/EVX Vehicle Model V2/Powertrain/Transmission Function ==
  data: T_FL output; Ratio input; T_FR output; T_RL output; Motor_Torque input; Splits input; T_RR output
function [T_FL,T_FR,T_RL,T_RR] = Transmission(Ratio,Motor_Torque,Splits)

T_FR = 0;
T_FL = T_FR;
T_RR = (Motor_Torque * Ratio) / (Splits + 1);
T_RL = T_RR;

== matlab function EVX_Lap_Simulation 2/EVX Vehicle Model V2/Subsystem/Car Parameters ==
  data: w output; m output; I output; kc output; cc output; h output
function [w,m,I,kc,cc,h] = Car_Param()

% Wheel Positions
a = 0.775;
b = 0.775;
d_F = 0.6;
e_F = 0.6;
d_R = 0.6;
e_R = 0.6;

w = [a,a,-b,-b;d_F,-e_F,d_R,-e_R];

% Mass & Intertias
m_WFL = 10;
m_WFR = 10;
m_WRL = 10;
m_WRR = 10;
m_c = 250;
m_cF = 125;
m_cR = m_c - m_cF;
I_cy = 50;
I_xF = 20;
I_xR = 20;
I_z = 50;

m = [m_WFL;m_WFR;m_WRL;m_WRR;m_c;m_cF;m_cR];
I = [I_cy;I_xF;I_xR;I_z];

% Chassis Stiffness
kc_x = 50000;

kc = [kc_x];

% Chassis Damping
cc_x = 500;

cc = [cc_x];

% Chassis COG Height
h_c = 0.3;
h_cF = 0.3;
h_cR = 0.3;

h = [h_c;h_cF;h_cR];

== matlab function EVX_Lap_Simulation 2/EVX Vehicle Model V2/Subsystem/Environment Parameters ==
  data: g output
function g  = Env_Param

g = -9.81;

== matlab function EVX_Lap_Simulation 2/EVX Vehicle Model V2/Tyre Model/MATLAB Function ==
  data: r input; F_x output; T input; F_x input
function F_x = Power_Lim(r,T,F_x)

max_F = T ./ r;

if T > 0
    for i = 1:4
        F_x(i) = min(F_x(i),max_F(i));
    end
end

if T < 0
    for i = 1:4
        F_x(i) = max(F_x(i),max_F(i));
    end
end

== matlab function EVX_Lap_Simulation 2/EVX Vehicle Model V2/Subsystem/Suspension Parameters ==
  data: kt output; ks output; kr output; ct output; cs output; cr output
function [kt,ks,kr,ct,cs,cr] = Sus_Param()

% Tyre Stiffness
kt_FL = 20000;
kt_FR = 20000;
kt_RL = 20000;
kt_RR = 20000;

kt = [kt_FL;kt_FR;kt_RL;kt_RR];

% Suspension Stiffness
ks_FL = 50000;
ks_FR = 50000;
ks_RL = 50000;
ks_RR = 50000;

ks = [ks_FL;ks_FR;ks_RL;ks_RR];

% Rollbar Stiffness
kr_Fx = 100;
kr_Rx = 100;
kr_Ly = 0;
kr_Ry = 0;
kr_FLRR = 0;
kr_FRRL = 0;

kr = [kr_Fx;kr_Rx;kr_Ly;kr_Ry;kr_FLRR;kr_FRRL];

% Tyre Damping
ct_FL = 250;
ct_FR = 250;
ct_RL = 250;
ct_RR = 250;

ct = [ct_FL;ct_FR;ct_RL;ct_RR];

% Suspension Damping
cs_FL = 250;
cs_FR = 250;
cs_RL = 250;
cs_RR = 250;

cs = [cs_FL;cs_FR;cs_RL;cs_RR];

% Rollbar Damping
cr_Fx = 25;
cr_Rx = 25;
cr_Ly = 0;
cr_Ry = 0;
cr_FLRR = 0;
cr_FRRL = 0;

cr = [cr_Fx;cr_Rx;cr_Ly;cr_Ry;cr_FLRR;cr_FRRL];

== matlab function EVX_Lap_Simulation 2/EVX Vehicle Model V2/Tyre Model/Slip Angle ==
  data: v_xw input; v_yw input; SA output; S input
function SA  = Slip_Angle(v_xw,v_yw,S)

% v_xw(v_xw == 0) = 0.001;

alpha = atand(v_yw ./ v_xw);

SA = S - alpha;

SA(v_yw == 0 & v_xw == 0) = 0;
SA(SA > 30) = 30;
SA(SA < -30) = -30;

== matlab function EVX_Lap_Simulation 2/EVX Vehicle Model V2/Tyre Model/Slip Ratio ==
  data: r input; dwheel input; v_xw input; SL output
function SL  = Slip_Ratio(r,dwheel,v_xw)

% v_xw(v_xw == 0) = 0.001;

SL = (((dwheel .* r) - v_xw) ./ abs(v_xw));

%limits on SL
SL(dwheel == 0 & v_xw == 0) = 0;
SL(dwheel > 0 & v_xw == 0) = 1;
SL(dwheel < 0 & v_xw == 0) = -1;
SL(SL > 1) = 1;
SL(SL < -1) = -1;

== matlab function EVX_Lap_Simulation 2/EVX Vehicle Model V2/Subsystem/Wheel Parameters ==
  data: r output; I output
function [r,I] = fcn()

r_FL = 0.175;
r_FR = 0.175;
r_RL = 0.175;
r_RR = 0.175;

I_FL = 5;
I_FR = 5;
I_RL = 5;
I_RR = 5;

r = [r_FL;r_FR;r_RL;r_RR];
I = [I_FL;I_FR;I_RL;I_RR];

== matlab function EVX_Lap_Simulation 2/EVX Vehicle Model V2/Powertrain/Brake Function ==
  data: v_wx input; Pedal input; Torque output
function Torque = fcn(v_wx,Pedal)

max_T = [1000;1000;1000;1000];

Torque = max_T .* Pedal/100 .* sign(v_wx);

== matlab function EVX_Lap_Simulation 2/EVX Vehicle Model V2/Tyre Model/Pacejka Tyre Model/MATLAB Function4 ==
  data: F_x output; SA input; F_y output; SL input; Fz input; M_z output
function [F_x,F_y,M_z] = Pacejka4(SA,SL,Fz)
SL = SL .* 30;
SM = sqrt(SA.^2 + SL.^2);
B = 18.6206;
C = 0.0180;
D = 3.5223e+04.*(-Fz./180).*0.6;
E = 1.1095;
F = zeros(length(D),1);
for i = 1:length(D)
D2 = D(i);
Sv = 0; %Vertical shift
Sh = 0; %Horizontal shift

x = 0.0174533.*SM(i) + Sh;
y = D2*sin(C*atan(B*x - E*(B*x - atan(B*x))));
F(i) = y + Sv;
end
theta = atand(SL./SA);
F_x = abs(F.*sind(theta)).*sign(SL);
F_y = abs(F.*cosd(theta)).*sign(SA);
M_z = zeros(size(SA));
F_x(isnan(F_x)) = 0;
F_y(isnan(F_y)) = 0;
M_z(isnan(M_z)) = 0;
end

== matlab function EVX_Lap_Simulation 2/EVX Vehicle Model V2/Horizontal Dynamics/Acceleration Forces ==
  data: a_x input; a_y input; ddtheta_z input; m input; h input; w input; M_y output; M_xF output; M_xR output
function [M_y,M_xF,M_xR] = fcn(a_x,a_y,ddtheta_z,m,h,w)

M_y = -m(5) * a_x * h(1);

a_yF = a_y + w(1,1)/2 * ddtheta_z;
a_yR = a_y + w(1,3)/2 * ddtheta_z;

M_xF = m(6) * a_yF * h(2);
M_xR = m(7) * a_yR * h(3);

== matlab function EVX_Lap_Simulation 2/EVX Vehicle Model V2/Horizontal Dynamics/Tyre_Forces1 ==
  data: F_Tx input; F_x output; F_Ty input; M_Tz input; S input; w input; F_y output; M_z output
function [F_x,F_y,M_z] = Tyre_Forces(F_Tx,F_Ty,M_Tz,S,w)

F_x = F_Tx(1) * cosd(S(1)) - F_Ty(1) * sind(S(1))...
    + F_Tx(2) * cosd(S(2)) - F_Ty(2) * sind(S(2))...
    + F_Tx(3) * cosd(S(3)) - F_Ty(3) * sind(S(3))...
    + F_Tx(4) * cosd(S(4)) - F_Ty(4) * sind(S(4));

F_y = F_Tx(1) * sind(S(1)) + F_Ty(1) * cosd(S(1))...
    + F_Tx(2) * sind(S(2)) + F_Ty(2) * cosd(S(2))...
    - F_Tx(3) * sind(S(3)) - F_Ty(3) * cosd(S(3))...
    - F_Tx(4) * sind(S(4)) - F_Ty(4) * cosd(S(4));

M_z = F_Tx(1) * (w(1,1) * sind(S(1)) - w(2,1) * cosd(S(1)))...
    + F_Ty(1) * (w(2,1) * sind(S(1)) + w(1,1) * cosd(S(1)))...
    + F_Tx(2) * (w(1,2) * sind(S(2)) - w(2,2) * cosd(S(2)))...
    + F_Ty(2) * (w(2,2) * sind(S(2)) + w(1,2) * cosd(S(2)))...
    + F_Tx(3) * (-w(1,3) * sind(S(3)) - w(2,3) * cosd(S(3)))...
    + F_Ty(3) * (w(2,3) * sind(S(3)) - w(1,3) * cosd(S(3)))...
    + F_Tx(4) * (-w(1,4) * sind(S(4)) - w(2,4) * cosd(S(4)))...
    + F_Ty(4) * (w(2,4) * sind(S(4)) - w(1,4) * cosd(S(4)))...
    - M_Tz(1) - M_Tz(2) + M_Tz(3) + M_Tz(4);
